simulink model "lab2"  (R2024a)
settings: Solver=VariableStepAuto  StartTime=0.0  StopTime=20  RelTol=1e-3
libraries: dspsrcs4 x2
settings Model: Creator=Adriana  LastModifiedBy=Adriana

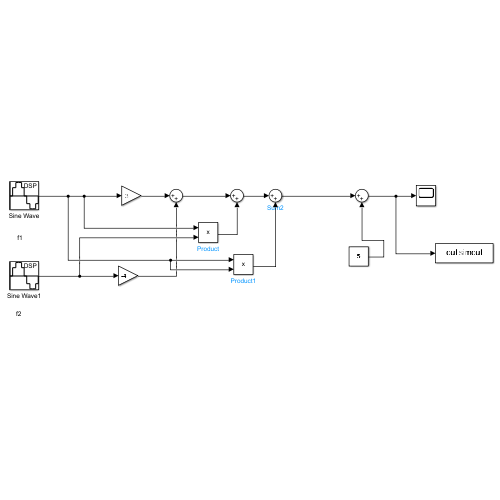
[thumbnail: Simulink's stored preview of the top-level diagram]
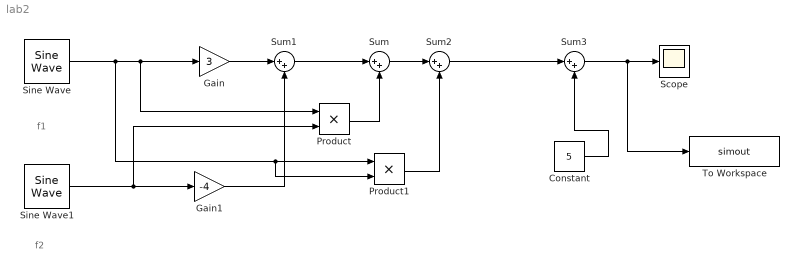
== system lab2 ==
  note: f2
  note: f1
  Constant : Constant  Value=5
  Gain : Gain  Gain=3
  Gain1 : Gain  Gain=-4
  Product : Product
  Product1 : Product
  Scope : Scope
  Sine Wave : dspsrcs4/Sine Wave  Amplitude=1  Frequency=1  Phase=0  SampleMode=Discrete  OutComplex=Real  CompMethod=Trigonometric fcn  TableSize=Speed  SampleTime=1/1000  SamplesPerFrame=1  ResetState=Restart at time zero  OutputFrames=off  dataType=double  wordLen=16  udDataType=sfix(16)  fracBitsMode=Best precision  numFracBits=15  OutDataTypeStr=double  LastOutDataTypeStr=double
  Sine Wave1 : dspsrcs4/Sine Wave  Amplitude=2  Frequency=0.1  Phase=pi/2  SampleMode=Discrete  OutComplex=Real  CompMethod=Trigonometric fcn  TableSize=Speed  SampleTime=1/1000  SamplesPerFrame=1  ResetState=Restart at time zero  OutputFrames=off  dataType=double  wordLen=16  udDataType=sfix(16)  fracBitsMode=Best precision  numFracBits=15  OutDataTypeStr=double  LastOutDataTypeStr=double
  Sum{,1..3} (4 alike) : Sum  Inputs=|++
  To Workspace : ToWorkspace  VariableName=simout  SaveFormat=Timeseries  SampleTime=-1
  wires:
  Sum2/1 -> Sum3/1
  Sine Wave/1 -> Product1/2, Product1/1, Product/1, Gain/1
  Sine Wave1/1 -> Product/2, Gain1/1
  Gain/1 -> Sum1/1
  Gain1/1 -> Sum1/2
  Sum1/1 -> Sum/1
  Product/1 -> Sum/2
  Sum/1 -> Sum2/1
  Constant/1 -> Sum3/2
  Product1/1 -> Sum2/2
  Sum3/1 -> To Workspace/1, Scope/1
